simulink model "Calcul_FT_Systeme_Simu"  (R2016a)
settings: Solver=VariableStepAuto  StartTime=0.0  StopTime=10.0  RelTol=1e-3
values from neighbouring files (symbols this model uses):
  K = K*0.97    (= 0.122115764944)    [Calcul_FT_Systeme.m]    (also in MethFreq.m = (10^(-A/20))/(Td*w))
  Te = 0.25    [Calcul_FT_Systeme.m]    (also in Modelisation_Mecanique.m = num(2,2)- num(1,2))
  Ti = Ti*0.4    (= 1.143)    [Calcul_FT_Systeme.m]    (also in MethFreq.m = 11.43/w)
undefined symbols (not defined in the file or in its folder): D_TFs, N_TFs
settings Model: Creator=charl  LastModifiedBy=charl

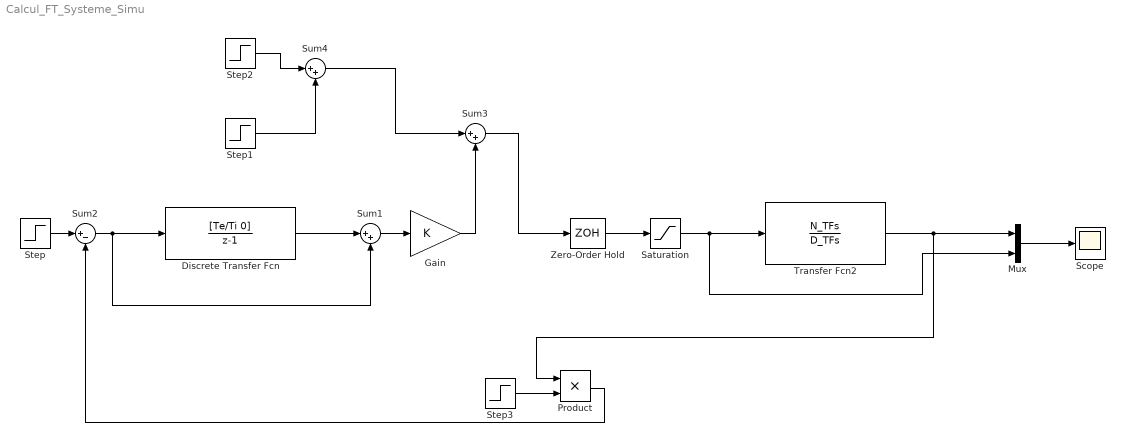
== system Calcul_FT_Systeme_Simu ==
  Discrete Transfer Fcn : DiscreteTransferFcn  Numerator=[Te/Ti 0]  Denominator=[1 -1]  SampleTime=Te
  Gain : Gain  Gain=K
  Mux : Mux  Inputs=2
  Product : Product
  Saturation : Saturate  UpperLimit=5  LowerLimit=0
  Scope : Scope
  Step : Step  Time=0  After=20  SampleTime=Te
  Step1 : Step  Time=0  After=0  SampleTime=Te
  Step2 : Step  Time=0  After=0  SampleTime=Te
  Step3 : Step  Time=0  SampleTime=Te
  Sum1 : Sum  Inputs=|++
  Sum2 : Sum  Inputs=|+-
  Sum3 : Sum  Inputs=|++
  Sum4 : Sum  Inputs=|++
  Transfer Fcn2 : TransferFcn  Numerator=N_TFs  Denominator=D_TFs
  Zero-Order Hold : ZeroOrderHold  SampleTime=Te
  wires:
  Zero-Order Hold/1 -> Saturation/1
  Discrete Transfer Fcn/1 -> Sum1/1
  Sum1/1 -> Gain/1
  Step/1 -> Sum2/1
  Sum2/1 -> Sum1/2, Discrete Transfer Fcn/1
  Mux/1 -> Scope/1
  Sum3/1 -> Zero-Order Hold/1
  Step2/1 -> Sum4/1
  Step1/1 -> Sum4/2
  Step3/1 -> Product/2
  Product/1 -> Sum2/2
  Transfer Fcn2/1 -> Product/1, Mux/1
  Gain/1 -> Sum3/2
  Sum4/1 -> Sum3/1
  Saturation/1 -> Transfer Fcn2/1, Mux/2
